simulink library "Load_lib"  (Simulink 8.1)
settings: Solver=ode45  StartTime=0.0  StopTime=10.0  RelTol=1e-3
undefined symbols (not defined in the file): gcbh, sps_rtmsupport
libraries: powerlib x1
settings Model: Creator=re25624  LastModifiedBy=ed12083

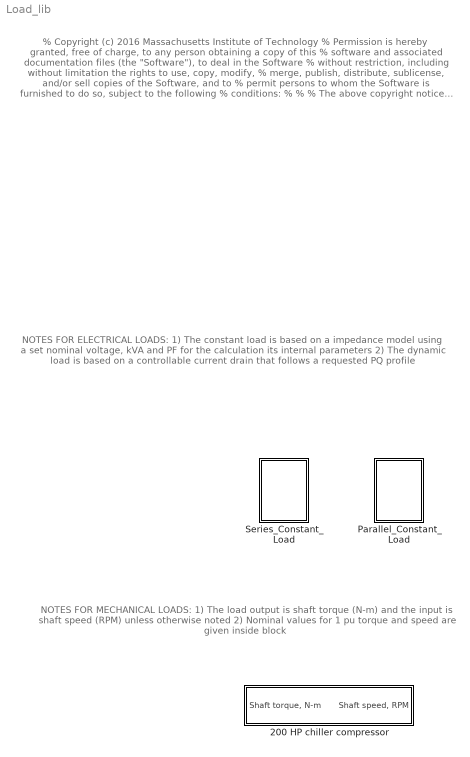
== system Load_lib ==
  note: NOTES FOR ELECTRICAL LOADS:
      | 1) The constant load is based on a impedance model using a set nominal voltage, kVA and PF for the calculation its internal parameters
      |
      | 2) The dynamic load is based on a controllable current drain that follows a requested PQ profile
  note: % Copyright (c) 2016 Massachusetts Institute of Technology
      | % Permission is hereby granted, free of charge, to any person obtaining a copy of this
      | % software and associated documentation files (the "Software"), to deal in the Software
      | % without restriction, including without limitation the rights to use, copy, modify,
      | % merge, publish, distribute, sublicense, and/or sell copies of the Software, and to
      | % permit persons to whom the Software is furnished to do so, subject to the following
      | % conditions:
      | %
      | %
      | % The above copyright notice and this permission notice shall be included in
      | % all copies or substantial portions of the Software.
      | %
      | % THE SOFTWARE IS PROVIDED "AS IS", WITHOUT WARRANTY OF ANY KIND, EXPRESS OR IMPLIED,
      | % INCLUDING BUT NOT LIMITED TO THE WARRANTIES OF MERCHANTABILITY, FITNESS FOR A
      | % PARTICULAR PURPOSE AND NONINFRINGEMENT. IN NO EVENT SHALL THE AUTHORS OR COPYRIGHT
      | % HOLDERS BE LIABLE FOR ANY CLAIM, DAMAGES OR OTHER LIABILITY, WHETHER IN AN ACTION
      | % OF CONTRACT, TORT OR OTHERWISE, ARISING FROM, OUT OF OR IN CONNECTION WITH THE
      | % SOFTWARE OR THE USE OR OTHER DEALINGS IN THE SOFTWARE.
      | %
      | %
      | %%
  note: NOTES FOR MECHANICAL LOADS:
      | 1) The load output is shaft torque (N-m) and the input is shaft speed (RPM) unless otherwise noted
      |
      | 2) Nominal values for 1 pu torque and speed are given inside block
  200 HP chiller compressor : Subsystem
  Parallel_Constant_Load : Subsystem  mask(Static Parallel PQ Load){v=460, kVA=100, pf=0.90}
      mask prompts: v "VRMSLL"
      mask help: The static load model is based on the default Simulink parallel load model. However, a mask was created to permit parametrization using nominal voltage, apparent power, and power factor.
  Series_Constant_Load : Subsystem  mask(Static Series PQ Load){v=460, kVA=100, pf=0.90}
      mask prompts: v "VRMSLL"
      mask help: The static load model is based on the default Simulink parallel load model. However, a mask was created to permit parametrization using nominal voltage, apparent power, and power factor.

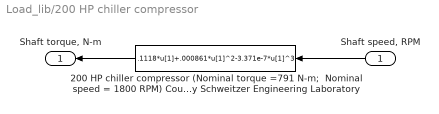
== system Load_lib/200 HP chiller compressor ==
  "Shaft speed, RPM" : Inport
  200 HP chiller compressor (Nominal torque =791 N-m;  Nominal speed = 1800 RPM) Courtesy Schweitzer Engineering Laboratory : Fcn  Expr=.1118*u[1]+.000861*u[1]^2-3.371e-7*u[1]^3
  "Shaft torque, N-m" : Outport
  wires:
  200 HP chiller compressor (Nominal torque =791 N-m;  Nominal speed = 1800 RPM) Courtesy Schweitzer Engineering Laboratory/1 -> "Shaft torque, N-m"/1
  "Shaft speed, RPM"/1 -> 200 HP chiller compressor (Nominal torque =791 N-m;  Nominal speed = 1800 RPM) Courtesy Schweitzer Engineering Laboratory/1

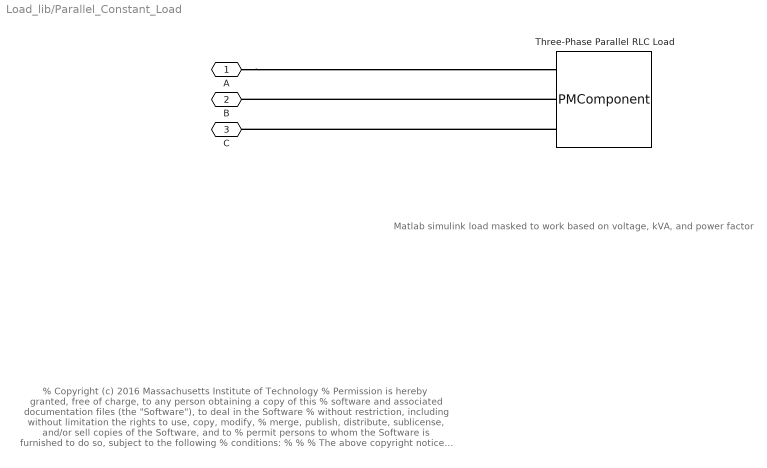
== system Load_lib/Parallel_Constant_Load ==
  note: Matlab simulink load masked to work based on voltage, kVA, and power factor
  note: % Copyright (c) 2016 Massachusetts Institute of Technology
      | % Permission is hereby granted, free of charge, to any person obtaining a copy of this
      | % software and associated documentation files (the "Software"), to deal in the Software
      | % without restriction, including without limitation the rights to use, copy, modify,
      | % merge, publish, distribute, sublicense, and/or sell copies of the Software, and to
      | % permit persons to whom the Software is furnished to do so, subject to the following
      | % conditions:
      | %
      | %
      | % The above copyright notice and this permission notice shall be included in
      | % all copies or substantial portions of the Software.
      | %
      | % THE SOFTWARE IS PROVIDED "AS IS", WITHOUT WARRANTY OF ANY KIND, EXPRESS OR IMPLIED,
      | % INCLUDING BUT NOT LIMITED TO THE WARRANTIES OF MERCHANTABILITY, FITNESS FOR A
      | % PARTICULAR PURPOSE AND NONINFRINGEMENT. IN NO EVENT SHALL THE AUTHORS OR COPYRIGHT
      | % HOLDERS BE LIABLE FOR ANY CLAIM, DAMAGES OR OTHER LIABILITY, WHETHER IN AN ACTION
      | % OF CONTRACT, TORT OR OTHERWISE, ARISING FROM, OUT OF OR IN CONNECTION WITH THE
      | % SOFTWARE OR THE USE OR OTHER DEALINGS IN THE SOFTWARE.
      | %
      | %
      | %%
  Three-Phase Parallel RLC Load : PMComponent  DialogController=POWERSYS.PowerSysDialog  LoadFcn=sps_rtmsupport('LoadFcn',gcbh);  StartFcn=sps_rtmsupport('StartFcn',gcbh);  StopFcn=sps_rtmsupport('StopFcn',gcbh);  PhysicalDomain=powersysdomain  LeftPortType=p1  RightPortType=p1  LConnTagsString=A|B|C  mask(Three-Phase Parallel RLC Load){Configuration=Y (grounded), NominalVoltage=v, NominalFrequency=60, ActivePower=kVA*1E3*pf, InductivePower=kVA*1E3*sqrt(1-pf^2), CapacitivePower=0, Measurements=None, LoadType=constant Z}
      mask prompts: NominalVoltage "Nominal phase-to-phase voltage Vn (Vrms)"; NominalFrequency "Nominal frequency fn (Hz):"; ActivePower "Active power P (W):"; InductivePower "Inductive reactive Power QL (positive var):"; CapacitivePower "Capacitive reactive power Qc (negative var):"; LoadType "Load type"
      mask help: Implements a three-phase parallel RLC load.
      mask init:
      | [s1,s2,s3,s4,r1,r2,l1,l2,c1,c2,c3,c4,x1,x2,x3,x4] = powericon('Parallel RLC Load',ActivePower,InductivePower,CapacitivePower);
      | ground = Configuration==1;
      | neutral = Configuration==3;
      | power_initmask();
      settings: AttributesFormatString=\n  CopyFcn=sps_rtmsupport('CopyFcn',gcbh);  DeleteFcn=sps_rtmsupport('DeleteFcn',gcbh);  UndoDeleteFcn=sps_rtmsupport('UndoDeleteFcn',gcbh);  ModelCloseFcn=sps_rtmsupport('ModelCloseFcn',gcbh);  PreSaveFcn=sps_rtmsupport('PreSaveFcn',gcbh);  PostSaveFcn=sps_rtmsupport('PostSaveFcn',gcbh);  NameChangeFcn=sps_rtmsupport('NameChangeFcn',gcbh);  PreCopyFcn=sps_rtmsupport('PreCopyFcn',gcbh);  OpenFcn=sps_rtmsupport('OpenFcn',gcbh, [1 7 8]);  CloseFcn=sps_rtmsupport('CloseFcn',gcbh);  PreDeleteFcn=sps_rtmsupport('PreDeleteFcn',gcbh);
      mask Help: helpview(psbhelp);
      mask TypeOptions Configuration: Y (grounded) | Y (floating) | Y (neutral) | Delta
      mask Callback Configuration: powericon('psbcallbacks',gcb,'Three-Phase Parallel RLC Load');
      mask TypeOptions Measurements: None | Branch voltages | Branch currents | Branch voltages and currents
      mask TypeOptions LoadType: constant Z | constant PQ
      mask Display:
      | plot(s1-50,s2,s3+30,s4,r1,r2,l1,l2,c1,c2,c3,c4,x1,x2,x3,x4)
      | 
      | plot( ground*[s3,s3],  ground*[-s2/4,s2/4])
      | plot( ground*[s3+10,s3+10], ground*[-s2/6,s2/6])
      | plot( ground*[s3+20,s3+20], ground*[-s2/10,s2/10])
      | 
      | plot( neutral*[ s3,s3+30], neutral*[0,0])
      | port_label('LConn', 1, 'A')
      | port_label('LConn', 2, 'B')
      | port_label('LConn', 3, 'C')
  A : PMIOPort  Port=1  Side=Right
  B : PMIOPort  Port=2  Side=Right
  C : PMIOPort  Port=3  Side=Right
  connections:
  Three-Phase Parallel RLC Load/LConn2 -- B/RConn1
  Three-Phase Parallel RLC Load/LConn3 -- C/RConn1
  A/RConn1 -- Three-Phase Parallel RLC Load/LConn1

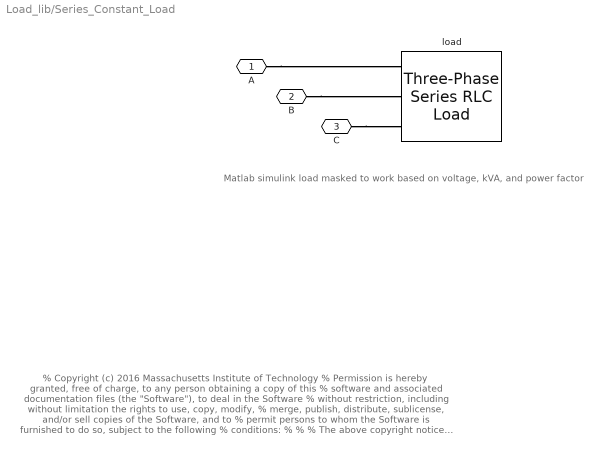
== system Load_lib/Series_Constant_Load ==
  note: Matlab simulink load masked to work based on voltage, kVA, and power factor
  note: % Copyright (c) 2016 Massachusetts Institute of Technology
      | % Permission is hereby granted, free of charge, to any person obtaining a copy of this
      | % software and associated documentation files (the "Software"), to deal in the Software
      | % without restriction, including without limitation the rights to use, copy, modify,
      | % merge, publish, distribute, sublicense, and/or sell copies of the Software, and to
      | % permit persons to whom the Software is furnished to do so, subject to the following
      | % conditions:
      | %
      | %
      | % The above copyright notice and this permission notice shall be included in
      | % all copies or substantial portions of the Software.
      | %
      | % THE SOFTWARE IS PROVIDED "AS IS", WITHOUT WARRANTY OF ANY KIND, EXPRESS OR IMPLIED,
      | % INCLUDING BUT NOT LIMITED TO THE WARRANTIES OF MERCHANTABILITY, FITNESS FOR A
      | % PARTICULAR PURPOSE AND NONINFRINGEMENT. IN NO EVENT SHALL THE AUTHORS OR COPYRIGHT
      | % HOLDERS BE LIABLE FOR ANY CLAIM, DAMAGES OR OTHER LIABILITY, WHETHER IN AN ACTION
      | % OF CONTRACT, TORT OR OTHERWISE, ARISING FROM, OUT OF OR IN CONNECTION WITH THE
      | % SOFTWARE OR THE USE OR OTHER DEALINGS IN THE SOFTWARE.
      | %
      | %
      | %%
  load : powerlib/Elements/Three-Phase Series RLC Load  LConnTagsString=A|B|C  Configuration=Y (grounded)  NominalVoltage=v  NominalFrequency=60  ActivePower=kVA*1E3*pf  InductivePower=kVA*1E3*sqrt(1-pf^2)  CapacitivePower=0  Measurements=None  LoadType=constant Z
  A : PMIOPort  Port=1  Side=Left
  B : PMIOPort  Port=2  Side=Left
  C : PMIOPort  Port=3  Side=Left
  connections:
  A/RConn1 -- load/LConn1
  B/RConn1 -- load/LConn2
  C/RConn1 -- load/LConn3
